simulink model "piddeneme"  (R2025b)
settings: Solver=VariableStepAuto  StartTime=0.0  StopTime=20.0  RelTol=1e-3
settings Model: Creator=halil  LastModifiedBy=halil

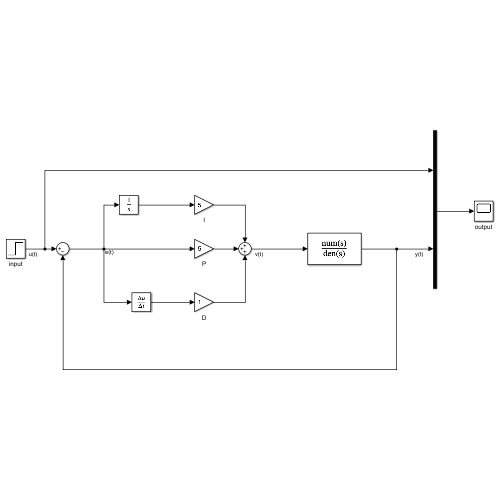
[thumbnail: Simulink's stored preview of the top-level diagram]
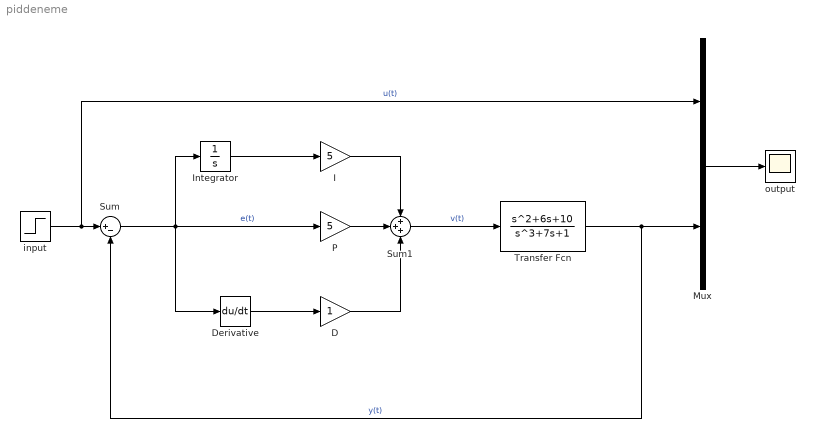
== system piddeneme ==
  D : Gain
  Derivative : Derivative
  I : Gain  Gain=5
  Integrator : Integrator
  Mux : Mux  Inputs=2
  P : Gain  Gain=5
  Sum : Sum  Inputs=|+-
  Sum1 : Sum  Inputs=+++
  Transfer Fcn : TransferFcn  Numerator=[1,6,10]  Denominator=[1,0,7,1]
  input : Step  SampleTime=0
  output : Scope
      settings: ActiveDisplayYMinimum=-0.13858737229642062  ActiveDisplayYMaximum=1.2472863506677858
  wires:
  Sum/1 -> Derivative/1, Integrator/1, P/1  "e(t)"
  Transfer Fcn/1 -> Mux/2, Sum/2  "y(t)"
  input/1 -> Mux/1, Sum/1  "u(t)"
  Sum1/1 -> Transfer Fcn/1  "v(t)"
  Mux/1 -> output/1
  Integrator/1 -> I/1
  P/1 -> Sum1/2
  I/1 -> Sum1/1
  Derivative/1 -> D/1
  D/1 -> Sum1/3
